simulink model "model2018"  (R2018b)
settings: Solver=VariableStepAuto  StartTime=0.0  StopTime=10  FixedStep=h  MaxStep=0.01  RelTol=1e-3
values from neighbouring files (symbols this model uses):
  angle_bound = [deg2rad(16.5),0,-deg2rad(13)]    [parameters.m]
  angle_real = [-0.0759,0.4e-3, 0.064]    [parameters.m]
  d_cart = 4.3726    [parameters.m]
  d_pend = 0.0097    [parameters.m]
  g = 9.81    [parameters.m]
  h = 0.01    [parameters.m]
  Km = 3.7228    [parameters.m]
  l = 0.6    [parameters.m]
  mc = 0.5477    [parameters.m]
  mp = 0.0760    (= 0.076)    [parameters.m]
  pend = [-0.573,-0.5590,-0.4870,-0.4180,-0.3530,-0.29,-0.225,-0.16,-0.094,-0.0247,-0.0037]    [parameters.m]
  sys = ss(A,B,C,D)    [linmod.m]
  ub_mtr_threshold = 0    [parameters.m]
  x_init = [0,0,0,0]    [parameters.m]
undefined symbols (not defined in the file or in its folder): adingain, adinoffs, Advantech, daoutgain, daoutoffs, K, PCI
libraries: cstblocks x3, sldrtlib x2, mpclib x1
settings Model: Creator=mdepo  LastModifiedBy=dvanhanswijk
settings DataIOCC: ReturnWorkspaceOutputs=on

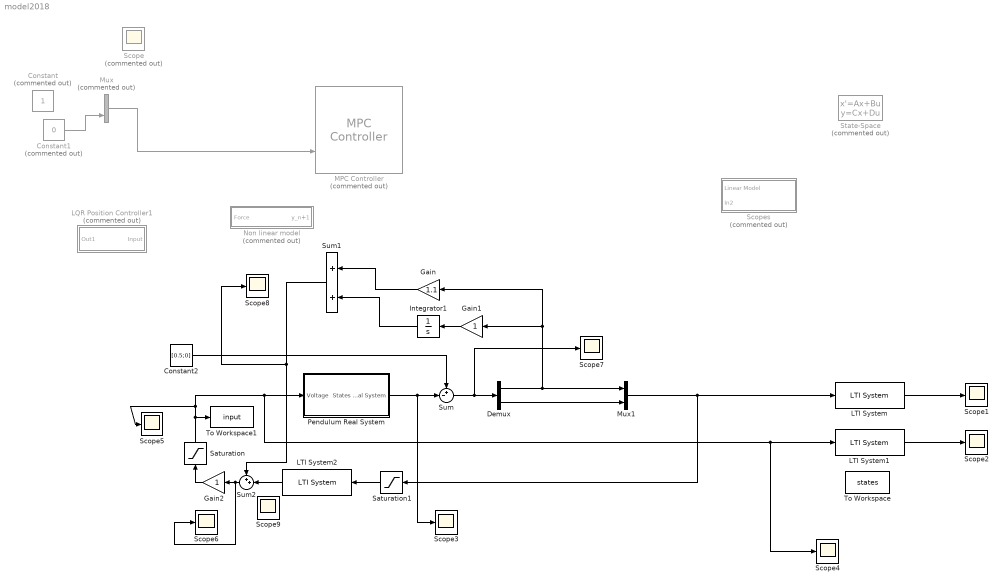
== system model2018 ==
  Constant : Constant  Commented=on
  Constant1 : Constant  Commented=on  Value=0
  Constant2 : Constant  Value=[0.5;0]
  Demux : Demux  Outputs=2
  Gain : Gain  Gain=1.1
  Gain1 : Gain
  Gain2 : Gain
  Integrator1 : Integrator
  LQR Position Controller1 : Subsystem  Commented=on
  LTI System : cstblocks/LTI System  sys=Ws  IC=[]
  LTI System1 : cstblocks/LTI System  sys=Wu  IC=[]
  LTI System2 : cstblocks/LTI System  sys=K  IC=[]
  MPC Controller : mpclib/MPC Controller  Commented=on  SCDEnableBlockLinearizationSpecification=on  mpcobj=mpcobj  is_multiple=0  enable_value=0  return_u0=off  updateMPCinCallerWorkspace=on  md_inport=off  mv_inport=off  return_cost=off  return_mvseq=off  return_qpstatus=off  return_xseq=off  return_state=off  return_ovseq=off  state_inport=off  umin_inport=off  umax_inport=off  ymin_inport=off  ymax_inport=off  cc_inport=off  ywt_inport=off  uwt_inport=off  duwt_inport=off  rhoeps_inport=off  uref_inport=off  n_ts=0.01  n_p=50  n_mv=1  n_md=0  n_ud=0  n_mo=1  n_uo=0  BlockDataType=double  SampleTimeInherited=off  switch_inport=off
      settings: SourceProductName=MATLAB Runtime - Model Predictive Control Toolbox Addin  SourceProductBaseCode=Missing
  Mux : Mux  Commented=on  Inputs=2
  Mux1 : Mux  Inputs=2
  Non linear model : Subsystem  Commented=on
  "Pendulum Real System " : Subsystem
  Saturation : Saturate  UpperLimit=1  LowerLimit=-1
  Saturation1 : Saturate  UpperLimit=100  LowerLimit=-100
  Scope : Scope  Commented=on
  Scope{1..9} (9 alike) : Scope
  "Scopes " : Subsystem  Commented=on
  State-Space : StateSpace  Commented=on  A=sys.A  B=sys.B  C=sys.C  D=sys.D  InitialCondition=x_init
  Sum : Sum  Inputs=+-|
  Sum1 : Sum  Inputs=|++
  Sum2 : Sum  Inputs=++|
  To Workspace : ToWorkspace  VariableName=states  SampleTime=h
  To Workspace1 : ToWorkspace  VariableName=input  SaveFormat=Timeseries  SampleTime=-1
  wires:
  Constant1/1 -> Mux/2
  Mux/1 -> MPC Controller/2
  LTI System/1 -> Scope1/1
  Constant2/1 -> Sum/1
  "Pendulum Real System "/1(States Real System) -> Sum/2, Scope3/1
  LTI System1/1 -> Scope2/1
  Sum2/1 -> Scope6/1, Gain2/1
  Sum/1 -> Scope7/1, Demux/1
  Demux/2 -> Mux1/2
  Mux1/1 -> Saturation1/1, LTI System/1
  Demux/1 -> Gain/1, Gain1/1, Mux1/1
  Gain1/1 -> Integrator1/1
  LTI System2/1 -> Sum2/2
  Sum1/1 -> Scope8/1, Sum2/1
  Integrator1/1 -> Sum1/2
  Gain/1 -> Sum1/1
  Gain2/1 -> Saturation/1
  Saturation1/1 -> LTI System2/1
  Saturation/1 -> Scope5/1, "Pendulum Real System "/1(Voltage), Scope4/1, LTI System1/1, To Workspace1/1

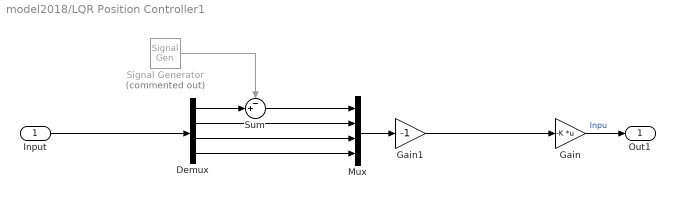
== system model2018/LQR Position Controller1 ==
  Input : Inport
  Demux : Demux
  Gain : Gain  Gain=-K  Multiplication=Matrix(K*u)
  Gain1 : Gain  Gain=-1
  Mux : Mux
  Signal Generator : SignalGenerator  Commented=on  Units=rad/sec
  Sum : Sum  Inputs=-+|
  Out1 : Outport
  wires:
  Signal Generator/1 -> Sum/1
  Sum/1 -> Mux/1
  Demux/1 -> Sum/2
  Mux/1 -> Gain1/1
  Input/1 -> Demux/1
  Demux/4 -> Mux/4
  Demux/3 -> Mux/3
  Demux/2 -> Mux/2
  Gain/1 -> Out1/1  "Inpu"
  Gain1/1 -> Gain/1

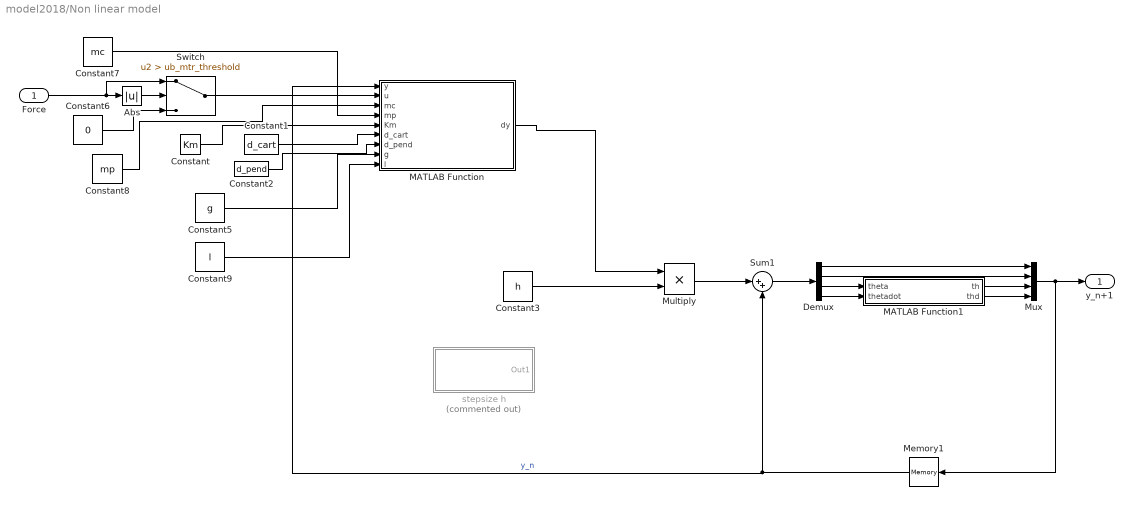
== system model2018/Non linear model ==
  Force : Inport
  Abs : Abs
  Constant : Constant  Value=Km
  Constant1 : Constant  Value=d_cart
  Constant2 : Constant  Value=d_pend
  Constant3 : Constant  Value=h  SampleTime=h
  Constant5 : Constant  Value=g
  Constant6 : Constant  Value=0
  Constant7 : Constant  Value=mc
  Constant8 : Constant  Value=mp
  Constant9 : Constant  Value=l
  Demux : Demux
  MATLAB Function : MATLAB Function  TreatAsAtomicUnit=on
  MATLAB Function1 : MATLAB Function  TreatAsAtomicUnit=on
  Memory1 : Memory  InitialCondition=x_init
  Multiply : Product
  Mux : Mux
  Sum1 : Sum  Inputs=|++
  Switch : Switch  Criteria=u2 > Threshold  Threshold=ub_mtr_threshold
  stepsize h : Subsystem  Commented=on
  y_n+1 : Outport
  wires:
  Abs/1 -> Switch/2
  Constant5/1 -> MATLAB Function/8(g)
  Constant6/1 -> Switch/3
  Sum1/1 -> Demux/1
  Mux/1 -> Memory1/1, y_n+1/1
  Constant3/1 -> Multiply/2
  Constant2/1 -> MATLAB Function/7(d_pend)
  Constant/1 -> MATLAB Function/5(Km)
  Memory1/1 -> MATLAB Function/1(y), Sum1/2  "y_n"
  MATLAB Function/1(dy) -> Multiply/1
  Demux/2 -> Mux/2
  Constant1/1 -> MATLAB Function/6(d_cart)
  Demux/1 -> Mux/1
  Force/1 -> Abs/1, Switch/1
  Multiply/1 -> Sum1/1
  Switch/1 -> MATLAB Function/2(u)
  Constant8/1 -> MATLAB Function/3(mc)
  Constant7/1 -> MATLAB Function/4(mp)
  Constant9/1 -> MATLAB Function/9(l)
  Demux/4 -> MATLAB Function1/2(thetadot)
  Demux/3 -> MATLAB Function1/1(theta)
  MATLAB Function1/1(th) -> Mux/3
  MATLAB Function1/2(thd) -> Mux/4

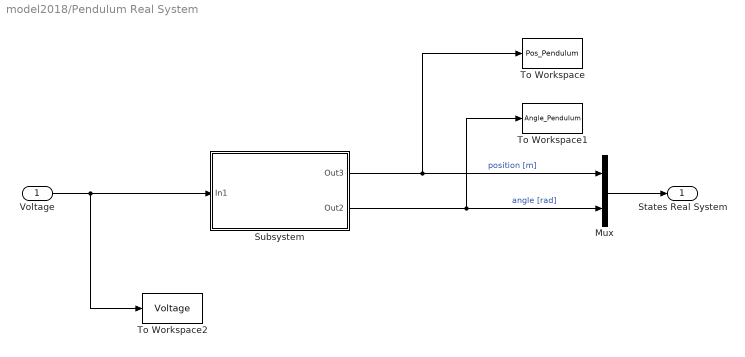
== system model2018/Pendulum Real System  ==
  Voltage : Inport
  Mux : Mux  Inputs=2
  Subsystem : Subsystem  InitFcn=hwinit  StartFcn=hwinit  mask{h=h}
      mask prompts: h "Sample time"
      mask init:
      | hwinit
      mask Display: disp('Pendulum');
  To Workspace : ToWorkspace  VariableName=Pos_Pendulum  SaveFormat=Timeseries  SampleTime=-1
  To Workspace1 : ToWorkspace  VariableName=Angle_Pendulum  SaveFormat=Timeseries  SampleTime=-1
  To Workspace2 : ToWorkspace  VariableName=Voltage  SaveFormat=Timeseries  SampleTime=-1
  States Real System : Outport
  wires:
  Voltage/1 -> To Workspace2/1, Subsystem/1(In1)
  Subsystem/1(Out3) -> To Workspace/1, Mux/1  "position [m]"
  Subsystem/2(Out2) -> Mux/2, To Workspace1/1  "angle [rad]"
  Mux/1 -> States Real System/1

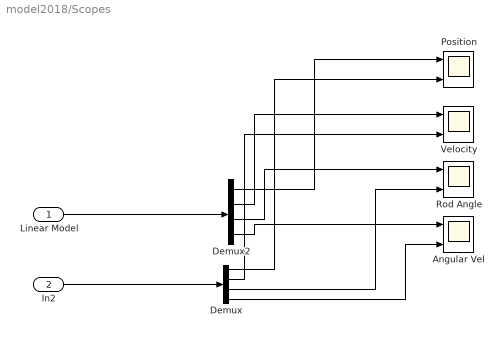
== system model2018/Scopes  ==
  Linear Model : Inport
  In2 : Inport  Port=2
  "Angular Vel " : Scope  NumInputPorts=2
  Demux : Demux
  Demux2 : Demux
  Position : Scope  NumInputPorts=2
  Rod Angle : Scope  NumInputPorts=2
  Velocity : Scope  NumInputPorts=2
  wires:
  Linear Model/1 -> Demux2/1
  Demux2/1 -> Position/1
  Demux2/2 -> Velocity/1
  Demux2/3 -> Rod Angle/1
  Demux2/4 -> "Angular Vel "/1
  In2/1 -> Demux/1
  Demux/1 -> Position/2
  Demux/2 -> Velocity/2
  Demux/3 -> Rod Angle/2
  Demux/4 -> "Angular Vel "/2

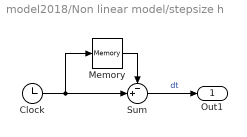
== system model2018/Non linear model/stepsize h ==
  Clock : Clock
  Memory : Memory
  Sum : Sum  Inputs=-+|
  Out1 : Outport
  wires:
  Memory/1 -> Sum/1
  Sum/1 -> Out1/1  "dt"
  Clock/1 -> Memory/1, Sum/2

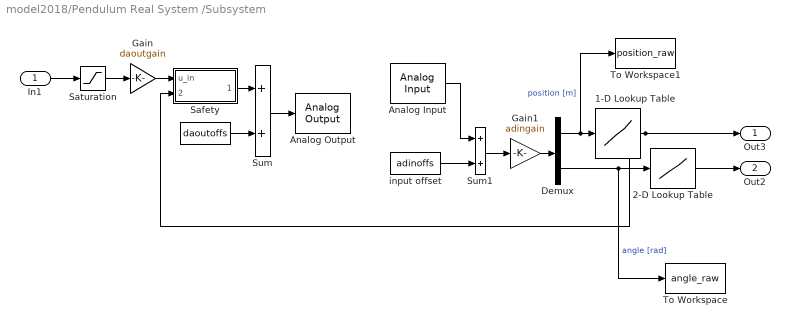
== system model2018/Pendulum Real System /Subsystem ==
  In1 : Inport
  " " : Constant  Value=daoutoffs
  1-D Lookup Table : Lookup_n-D  NumberOfTableDimensions=1  BreakpointsForDimension1=pend  Table=real  InternalRulePriority=Speed  RndMeth=Simplest  InputSameDT=on
  2-D Lookup Table : Lookup_n-D  NumberOfTableDimensions=1  BreakpointsForDimension1=angle_real  BreakpointsForDimension2=[1:3]  Table=angle_bound  InternalRulePriority=Speed  RndMeth=Simplest  InputSameDT=on
  Analog Input : sldrtlib/Analog Input  SampleTime=h  MaxMissedTicks=ticklost  ShowMissedTicks=off  YieldWhenWaiting=on  DrvName=Advantech/PCI-1711  DrvAddress=4294967295  DrvOptions=zeros(1,0)  Channels=adinchannels  RangeMode=2  VoltRange=1  DataType=1
      settings: AttributesFormatString=Advantech\nPCI-1711 [auto]  SourceProductName=Simulink Desktop Real-Time
  Analog Output : sldrtlib/Analog Output  SampleTime=h  MaxMissedTicks=ticklost  ShowMissedTicks=off  YieldWhenWaiting=off  DrvName=Advantech/PCI-1711  DrvAddress=4294967295  DrvOptions=zeros(1,0)  Channels=daoutchannels  RangeMode=2  VoltRange=2  InitialValue=0  FinalValue=0
      settings: AttributesFormatString=Advantech\nPCI-1711 [auto]  SourceProductName=Simulink Desktop Real-Time
  Demux : Demux  Outputs=2
  Gain : Gain  Gain=daoutgain  SaturateOnIntegerOverflow=on  OutDataTypeStr=Inherit: Same as input  ParamDataTypeStr=Inherit: Same as input
  Gain1 : Gain  Gain=adingain  SaturateOnIntegerOverflow=on  OutDataTypeStr=Inherit: Same as input  ParamDataTypeStr=Inherit: Same as input
  Safety : Subsystem
      mask help: The output of the block is restricted to prevent damage to the system. If the cart reaches some safety margins (left: -0.26 and right: 0.26), the output of the block is nullifed. Then the control has to be restarted.
      mask Display: disp('Safety \n margins')
  Saturation : Saturate  UpperLimit=1  LowerLimit=-1
  Sum : Sum  SaturateOnIntegerOverflow=on  OutDataTypeStr=Inherit: Same as first input
  Sum1 : Sum  SaturateOnIntegerOverflow=on  InputSameDT=on  OutDataTypeStr=Inherit: Same as first input
  To Workspace : ToWorkspace  VariableName=angle_raw  SaveFormat=Timeseries  SampleTime=-1
  To Workspace1 : ToWorkspace  VariableName=position_raw  SaveFormat=Timeseries  SampleTime=-1
  input offset : Constant  Value=adinoffs
  Out3 : Outport
  Out2 : Outport  Port=2
  wires:
  Sum1/1 -> Gain1/1
  input offset/1 -> Sum1/2
  Analog Input/1 -> Sum1/1
  Gain1/1 -> Demux/1
  Saturation/1 -> Gain/1
  Sum/1 -> Analog Output/1
  " "/1 -> Sum/2
  In1/1 -> Saturation/1
  Demux/2 -> 2-D Lookup Table/1, To Workspace/1  "angle [rad]"
  Safety/1(u_out) -> Sum/1
  Gain/1 -> Safety/1(u_in)
  Demux/1 -> To Workspace1/1, 1-D Lookup Table/1  "position [m]"
  1-D Lookup Table/1 -> Safety/2(Position), Out3/1
  2-D Lookup Table/1 -> Out2/1

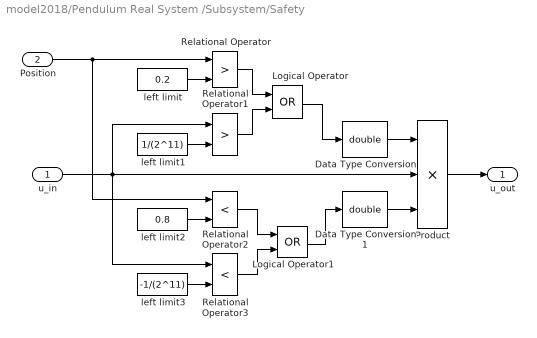
== system model2018/Pendulum Real System /Subsystem/Safety ==
  u_in : Inport
  Position : Inport  Port=2
  Data Type Conversion : DataTypeConversion  OutDataTypeStr=double
  Data Type Conversion1 : DataTypeConversion  OutDataTypeStr=double
  Logical Operator : Logic  Operator=OR  OutDataTypeStr=boolean
  Logical Operator1 : Logic  Operator=OR  OutDataTypeStr=boolean
  Product : Product  Inputs=3  SaturateOnIntegerOverflow=on  InputSameDT=on  OutDataTypeStr=Inherit: Same as first input
  Relational Operator : RelationalOperator  Operator=>  OutDataTypeStr=boolean  RndMeth=Nearest  InputSameDT=on
  Relational Operator1 : RelationalOperator  Operator=>  OutDataTypeStr=boolean  RndMeth=Nearest  InputSameDT=on
  Relational Operator2 : RelationalOperator  Operator=<  OutDataTypeStr=boolean  RndMeth=Nearest  InputSameDT=on
  Relational Operator3 : RelationalOperator  Operator=<  OutDataTypeStr=boolean  RndMeth=Nearest  InputSameDT=on
  left limit : Constant  Value=0.2
  left limit1 : Constant  Value=1/(2^11)
  left limit2 : Constant  Value=0.8
  left limit3 : Constant  Value=-1/(2^11)
  u_out : Outport
  wires:
  left limit1/1 -> Relational Operator1/2
  u_in/1 -> Relational Operator1/1, Relational Operator3/1, Product/2
  Logical Operator1/1 -> Data Type Conversion1/1
  Logical Operator/1 -> Data Type Conversion/1
  left limit/1 -> Relational Operator/2
  Relational Operator/1 -> Logical Operator/1
  Relational Operator1/1 -> Logical Operator/2
  Position/1 -> Relational Operator/1, Relational Operator2/1
  left limit2/1 -> Relational Operator2/2
  Relational Operator2/1 -> Logical Operator1/1
  left limit3/1 -> Relational Operator3/2
  Relational Operator3/1 -> Logical Operator1/2
  Product/1 -> u_out/1
  Data Type Conversion/1 -> Product/1
  Data Type Conversion1/1 -> Product/3

== matlab function model2018/Non linear model/MATLAB Function1 ==
  data: theta input; th output; thetadot input; thd output
function [th,thd] = fcn(theta, thetadot)

threshold = 0.26;

if abs(theta) > threshold
    th = threshold;
    thd = 0;
else
    th = theta;
    thd = thetadot;
end

== matlab function model2018/Non linear model/MATLAB Function ==
  data: y input; u input; dy output; mc input; mp input; Km input; d_cart input; d_pend input; g input; l input
function dy = fcn(y,u,mc,mp,Km,d_cart,d_pend,g,l)
dy = zeros(4,1);
dy(1,1) = y(2);
dy(2,1) = 1/((mc+mp)*(1-0.75*mp))*(Km*u - d_cart*y(2) + 3/(2*l)*((l/2)*mp*g*y(3) - d_pend*y(4)) + 0*mp*l*y(4)^2*y(3)/2);
dy(3,1) = y(4);
dy(4,1) = 3/(mp*l^2)*(l*mp*dy(2,1)/2 + l*mp*g*y(3)/2 - d_pend*y(4));
end
